simulink model "Lab6_aproks"  (R2017a)
settings: Solver=FixedStepAuto  StartTime=0.0  StopTime=10.0  FixedStep=0.1  RelTol=1e-3
libraries: cstblocks x2
settings Model: Creator=ishiguro  LastModifiedBy=ishiguro
settings DataIOCC: TimeSaveName=tout_aproks

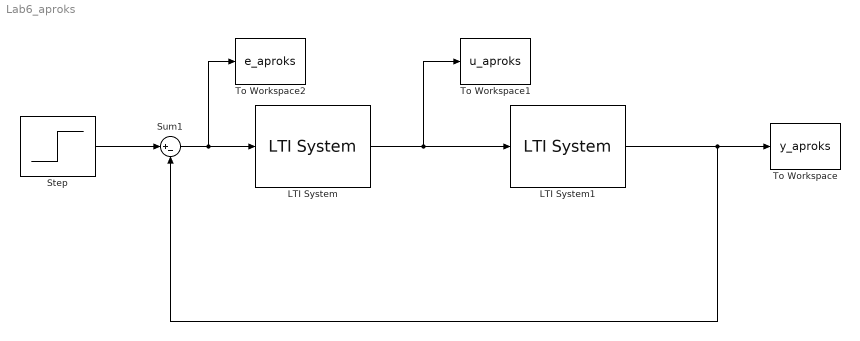
== system Lab6_aproks ==
  LTI System : cstblocks/LTI System  sys=kL  IC=[]
  LTI System1 : cstblocks/LTI System  sys=L  IC=[]
  Step : Step  Time=0  SampleTime=0
  Sum1 : Sum  Inputs=|+-
  To Workspace : ToWorkspace  VariableName=y_aproks  SampleTime=-1
  To Workspace1 : ToWorkspace  VariableName=u_aproks  SampleTime=-1
  To Workspace2 : ToWorkspace  VariableName=e_aproks  SampleTime=-1
  wires:
  Sum1/1 -> To Workspace2/1, LTI System/1
  Step/1 -> Sum1/1
  LTI System/1 -> To Workspace1/1, LTI System1/1
  LTI System1/1 -> To Workspace/1, Sum1/2
